simulink model "parameter_sweep_Mechanical"  (R2020a)
settings: Solver=FixedStepAuto  StartTime=0.0  StopTime=0.05  FixedStep=0.00001  RelTol=1e-3
values from neighbouring files (symbols this model uses):
  A_w = 1    [parameter_sweep_LRM_plotter.m]    (also in parameter_sweep_Mechanical_plotter.m)
  D_V = 0.00001    (= 1e-05)    [parameter_sweep_Mechanical_plotter.m]
  F_BW = 0.00001    (= 1e-05)    [parameter_sweep_Mechanical_plotter.m]
  F_C = 0.00001    (= 1e-05)    [parameter_sweep_Mechanical_plotter.m]
  G = -(Mass * 9.81)    (= -0.3924)    [parameter_sweep_Mechanical_plotter.m]
  K = 0.25    [parameter_sweep_Mechanical_plotter.m]
  K_Z = 0    [parameter_sweep_Mechanical_plotter.m]
  l_w = 1    [parameter_sweep_LRM_plotter.m]    (also in parameter_sweep_Mechanical_plotter.m)
  Ltch_End = 15    [parameter_sweep_Mechanical_plotter.m]
  Ltch_St = 12    [parameter_sweep_Mechanical_plotter.m]
  Ltch_Str = 5    [parameter_sweep_Mechanical_plotter.m]
  Mass = 0.04    [parameter_sweep_Mechanical_plotter.m]
  Mur = 1    [parameter_sweep_Mechanical_plotter.m]
  Nw = 4    [parameter_sweep_LRM_plotter.m]    (also in parameter_sweep_Mechanical_plotter.m = 300)
  R = 4.95    [parameter_sweep_LRM_plotter.m]    (also in parameter_sweep_LR_plotter.m = 7; parameter_sweep_M_plotter.m = 7; parameter_sweep_Mechanical_plotter.m = 5)
  R_Int = 0.55    [parameter_sweep_LRM_plotter.m]    (also in parameter_sweep_Mechanical_plotter.m = 0.33)
  Rel = Nw^2/ (0.004)    (= 4000)    [parameter_sweep_LRM_plotter.m]    (also in parameter_sweep_M_plotter.m = 0 + ((i-1) * 10); parameter_sweep_Mechanical_plotter.m = 0)
  Rel2 = (Nw^2)/ (0.08)    (= 1125000)    [parameter_sweep_Mechanical_plotter.m]
  V_T = 33.5    [parameter_sweep_LRM_plotter.m]    (also in parameter_sweep_LR_plotter.m = 4 + ((i-1) * 1); parameter_sweep_M_plotter.m = 350; parameter_sweep_Mechanical_plotter.m)
undefined symbols (not defined in the file or in its folder): R_Rate
libraries: nesl_utility x29, fl_lib x20, simulink x3, sdl_lib x1
settings Model: Creator=insat  LastModifiedBy=gwb15193

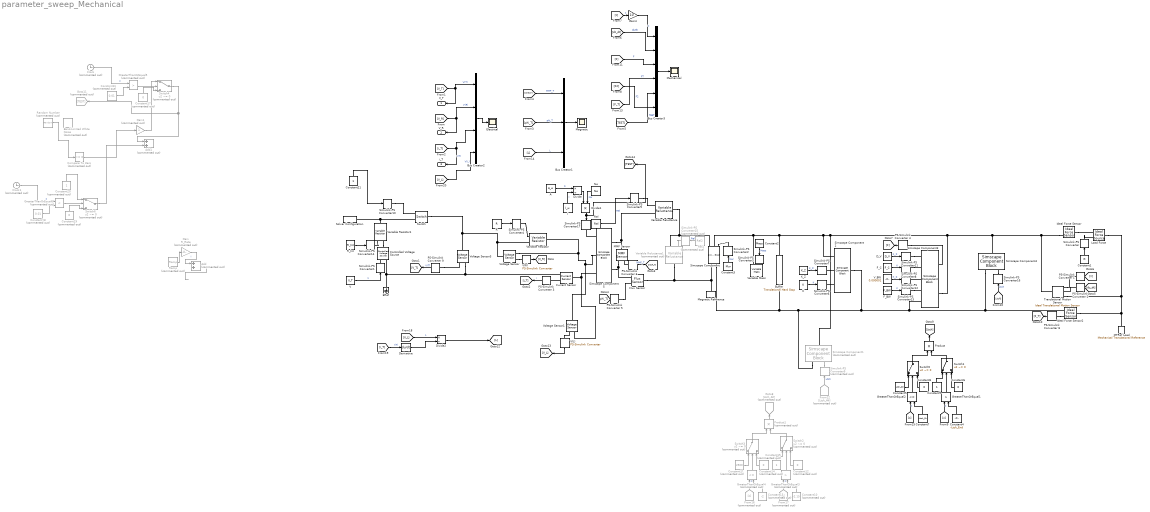
== system parameter_sweep_Mechanical ==
  A : Constant  Value=A_w
  Add : Sum  Commented=on
  Add1 : Sum  Commented=on
  Band-Limited White Noise : simulink/Sources/Band-Limited White Noise  Commented=on  Cov=[0.001]  Ts=0.00001  seed=[2334]
  Buffer : fl_lib/Mechanical/Translational Elements/Translational Hard Stop  upper_bnd=20 mm  lower_bnd=-.9 mm  stiff_up=100 N/mm  stiff_low=100 N/mm  D_up=10000000000000 s*N/mm  D_low=100 s*N/mm  model=simscape.enum.hardstop.fullundamped  transition=1 mm  v_specify=off  v_priority=None  v=0 m/s  v_nominal_specify=off  v_nominal_unit=m/s  v_nominal_value=1  f_specify=off  f_priority=None  f=0 N  f_nominal_specify=off  f_nominal_unit=N  f_nominal_value=1  x_specify=off  x_priority=High  x=0 m  x_nominal_specify=off  x_nominal_unit=m  x_nominal_value=1
  Bus Creator1 : BusCreator  Inputs=3
  Bus Creator2 : BusCreator  Inputs=4
  Bus Creator3 : BusCreator  Inputs=6
  Clock : Clock  Commented=on
  Clock1 : Clock  Commented=on
  Compare To Zero : simulink/Logic and Bit Operations/Compare To Zero  Commented=on  relop=<=  OutDataTypeStr=boolean
  Constant1 : Constant  Value=G
  Constant10 : Constant  Commented=on  Value=-2.15
  Constant11 : Constant  Commented=on  Value=2500
  Constant{12,14,17,19} (4 alike) : Constant  Commented=on  Value=0
  Constant13 : Constant  Commented=on  Value=-2
  Constant15 : Constant  Commented=on
  Constant16 : Constant  Commented=on  Value=0.01
  Constant18 : Constant  Commented=on  Value=0.01
  Constant2 : Constant  Value=Mass
  Constant20 : Constant  Commented=on
  Constant21 : Constant
  Constant3 : Constant  Value=Mur
  Constant4 : Constant  Value=-Ltch_End
  Constant5 : Constant  Value=Ltch_Str
  Constant6 : Constant  Value=0
  Constant7 : Constant  Value=-Ltch_St
  Constant8 : Constant  Value=0
  Constant9 : Constant
  Controlled Voltage Source : fl_lib/Electrical/Electrical Sources/Controlled Voltage Source
  Current Sensor : fl_lib/Electrical/Electrical Sensors/Current Sensor
  D_V : Constant  Value=D_V
  Derivative : Derivative
  Divide : Product  Inputs=*/
  Divide1 : Product  Inputs=**
  Divide2 : Product  Inputs=*/
  ERef : fl_lib/Electrical/Electrical Elements/Electrical Reference
  Electrical : Scope
  F_BW : Constant  Value=F_BW
  F_C : Constant  Value=F_C
  Flux Sensor : fl_lib/Magnetic/Magnetic Sensors/Flux Sensor
      settings: SourceProductBaseCode=SS  InternalSimscapePortConfiguration="{\"Bottom\":[],\"Left\":[{\"id\":\"N\",\"label\":\"N\",\"type\":\"foundation.magnetic.magnetic\"}],\"Right\":[{\"id\":\"PHI\",\"label\":\"\",\"type\":\"output\"},{\"id\":\"S\",\"label\":\"S\",\"type\":\"foundation.magnetic.magnetic\"}],\"Top\":[]}"
  From12 : From  Commented=on  GotoTag=Ltch_Alt
  From16 : From  Commented=on  GotoTag=z
  From17 : From  Commented=on  GotoTag=z
  Gain : Gain  Commented=on  Gain=R_Rate
  Gain1 : Gain  Commented=on
  Gain4 : Gain  Gain=10
  Goto11 : Goto  Commented=on  GotoTag=TEST
  Goto8 : Goto  Commented=on  GotoTag=Ltch_Alt
  GreaterThanOrEqual1 : RelationalOperator  Operator=>  OutDataTypeStr=boolean  ZeroCross=off  RndMeth=Simplest
  GreaterThanOrEqual2 : RelationalOperator  Operator=<=  OutDataTypeStr=boolean  ZeroCross=off  RndMeth=Simplest
  GreaterThanOrEqual3 : RelationalOperator  Commented=on  Operator=>  OutDataTypeStr=boolean  ZeroCross=off  RndMeth=Simplest
  GreaterThanOrEqual4 : RelationalOperator  Commented=on  Operator=<=  OutDataTypeStr=boolean  ZeroCross=off  RndMeth=Simplest
  GreaterThanOrEqual5 : RelationalOperator  Commented=on  Operator=>  OutDataTypeStr=boolean  ZeroCross=off  RndMeth=Simplest
  GreaterThanOrEqual6 : RelationalOperator  Commented=on  Operator=<  OutDataTypeStr=boolean  ZeroCross=off  RndMeth=Simplest
  Ideal Force Sensor : fl_lib/Mechanical/Mechanical Sensors/Ideal Force Sensor
  Ideal Force Sensor2 : fl_lib/Mechanical/Mechanical Sensors/Ideal Force Sensor
  K : Constant  Value=K
  K_Z : Constant  Value=K_Z
  Load Force : fl_lib/Mechanical/Mechanical Sources/Ideal Force Source
  MMF Sensor : fl_lib/Magnetic/Magnetic Sensors/MMF Sensor
      settings: SourceProductBaseCode=SS  InternalSimscapePortConfiguration="{\"Bottom\":[],\"Left\":[{\"id\":\"N\",\"label\":\"N\",\"type\":\"foundation.magnetic.magnetic\"}],\"Right\":[{\"id\":\"MMF\",\"label\":\"\",\"type\":\"output\"},{\"id\":\"S\",\"label\":\"S\",\"type\":\"foundation.magnetic.magnetic\"}],\"Top\":[]}"
  MTRef Load : fl_lib/Mechanical/Translational Elements/Mechanical Translational Reference
  Magnetic : Scope
  Magnetic Reference : fl_lib/Magnetic/Magnetic Elements/Magnetic Reference
      settings: SourceProductBaseCode=SS  InternalSimscapePortConfiguration="{\"Bottom\":[],\"Left\":[{\"id\":\"M\",\"label\":\"\",\"type\":\"foundation.magnetic.magnetic\"}],\"Right\":[],\"Top\":[]}"
  Mechanical : Scope
  Nw : Constant  Value=Nw
  PS-Simulink Converter 1 : nesl_utility/PS-Simulink Converter  PhysicalDomain=network_engine_domain  SubClassName=ps_output  LeftPortType=input  RightPortType=output  PseudoPeriodic=off  Frequencies=[]  Unit=mm  AffineConversion=off
  PS-Simulink Converter 2 : nesl_utility/PS-Simulink Converter  PhysicalDomain=network_engine_domain  SubClassName=ps_output  LeftPortType=input  RightPortType=output  PseudoPeriodic=off  Frequencies=[]  Unit=mm/s  AffineConversion=off
  PS-Simulink Converter 3 : nesl_utility/PS-Simulink Converter  PhysicalDomain=network_engine_domain  SubClassName=ps_output  LeftPortType=input  RightPortType=output  PseudoPeriodic=off  Frequencies=[]  Unit=A  AffineConversion=off
  PS-Simulink Converter 4 : nesl_utility/PS-Simulink Converter  PhysicalDomain=network_engine_domain  SubClassName=ps_output  LeftPortType=input  RightPortType=output  PseudoPeriodic=off  Frequencies=[]  Unit=N  AffineConversion=off
  PS-Simulink Converter 5 : nesl_utility/PS-Simulink Converter  PhysicalDomain=network_engine_domain  SubClassName=ps_output  LeftPortType=input  RightPortType=output  PseudoPeriodic=off  Frequencies=[]  Unit=Wb  AffineConversion=off
  PS-Simulink Converter 6 : nesl_utility/PS-Simulink Converter  PhysicalDomain=network_engine_domain  SubClassName=ps_output  LeftPortType=input  RightPortType=output  PseudoPeriodic=off  Frequencies=[]  Unit=A  AffineConversion=off
  PS-Simulink Converter 8 : nesl_utility/PS-Simulink Converter  PhysicalDomain=network_engine_domain  SubClassName=ps_output  LeftPortType=input  RightPortType=output  PseudoPeriodic=off  Frequencies=[]  Unit=N  AffineConversion=off
  PS-Simulink Converter 9 : nesl_utility/PS-Simulink Converter  PhysicalDomain=network_engine_domain  SubClassName=ps_output  LeftPortType=input  RightPortType=output  PseudoPeriodic=off  Frequencies=[]  Unit=V  AffineConversion=off
  Product : Product
  Product1 : Product  Commented=on
  R : Constant  Value=R
  R_Int : Constant  Value=R_Int
  Ramp : simulink/Sources/Ramp  Commented=on  slope=1  start=0.01  InitialOutput=0
  Random Number : RandomNumber  Commented=on  Mean=-30  Variance=1000  SampleTime=0.0001
  Rel : Constant  Value=Rel
  Rel1 : Constant  Commented=on  Value=Rel2
  Simscape Component : SimscapeComponentBlock  SourceFile=reluctance_force_actuator_modified  ComponentPath=reluctance_force_actuator_modified  ComponentVariants="[\"reluctance_force_actuator_modified\"]"  ComponentVariantNames="[\"reluctance_force_actuator_modified\"]"  ClassName=reluctance_force_actuator_modified  SchemaVersion=1  x0=22 mm  xbffr=1e-4 mm  CSA=1.7671 cm^2  K_contact=0.001 N/mm  D_contact=0.001 s*N/mm  mmf_specify=off  mmf_priority=None  mmf=0 A  mmf_nominal_specify=off  mmf_nominal_unit=A  mmf_nominal_value=1  phi_specify=off  phi_priority=None  phi=0 Wb  phi_nominal_specify=off  phi_nominal_unit=Wb  phi_nominal_value=1  f_specify=off  f_priority=None  f=0 N  f_nominal_specify=off  f_nominal_unit=N  f_nominal_value=1  u_specify=off  u_priority=None  u=0 m/s  u_nominal_specify=off  u_nominal_unit=m/s  u_nominal_value=1
      settings: CopyFcn=simscape.engine.sli.internal.componentblockcallback(gcbh,'COPY')  PreCopyFcn=simscape.engine.sli.internal.componentblockcallback(gcbh,'PRECOPY')  PreDeleteFcn=simscape.engine.sli.internal.componentblockcallback(gcbh,'PREDELETE')  InternalSimscapePortConfiguration="{\"Bottom\":[],\"Left\":[{\"id\":\"N\",\"label\":\"N\",\"type\":\"foundation.magnetic.magnetic\"},{\"id\":\"R\",\"label\":\"R\",\"type\":\"foundation.mechanical.translational.translational\"},{\"id\":\"mur\",\"label\":\"Mur\",\"type\":\"input\"}],\"Right\":[{\"id\":\"S\",\"label\":\"S\",\"type\":\"foundation.magnetic.magnetic\"},{\"id\":\"C\",\"label\":\"C\",\"type\":\"foundation.mechanical.translational.translational\"}],\"Top\":[]}"
      mask Type: Reluctance Force Actuator
  Simscape Component1 : SimscapeComponentBlock  Commented=on  SourceFile=damper_mod  ComponentPath=damper_mod  ComponentVariants="[\"damper_mod\"]"  ComponentVariantNames="[\"damper_mod\"]"  ClassName=damper_mod  SchemaVersion=1  v_specify=off  v_priority=None  v=0 m/s  v_nominal_specify=off  v_nominal_unit=m/s  v_nominal_value=1  f_specify=off  f_priority=None  f=0 N  f_nominal_specify=off  f_nominal_unit=N  f_nominal_value=1
      settings: CopyFcn=simscape.engine.sli.internal.componentblockcallback(gcbh,'COPY')  PreCopyFcn=simscape.engine.sli.internal.componentblockcallback(gcbh,'PRECOPY')  PreDeleteFcn=simscape.engine.sli.internal.componentblockcallback(gcbh,'PREDELETE')  InternalSimscapePortConfiguration="{\"Bottom\":[],\"Left\":[{\"id\":\"R\",\"label\":\"R\",\"type\":\"foundation.mechanical.translational.translational\"},{\"id\":\"D\",\"label\":\"Damping coefficient\",\"type\":\"input\"}],\"Right\":[{\"id\":\"C\",\"label\":\"C\",\"type\":\"foundation.mechanical.translational.translational\"}],\"Top\":[]}"
      mask Type: Translational Damper
  Simscape Component2 : SimscapeComponentBlock  SourceFile=var_trans_spring_mod  ComponentPath=var_trans_spring_mod  ComponentVariants="[\"var_trans_spring_mod\"]"  ComponentVariantNames="[\"var_trans_spring_mod\"]"  ClassName=var_trans_spring_mod  SchemaVersion=1  Kmin=1 N/m
      settings: CopyFcn=simscape.engine.sli.internal.componentblockcallback(gcbh,'COPY')  PreCopyFcn=simscape.engine.sli.internal.componentblockcallback(gcbh,'PRECOPY')  PreDeleteFcn=simscape.engine.sli.internal.componentblockcallback(gcbh,'PREDELETE')  InternalSimscapePortConfiguration="{\"Bottom\":[],\"Left\":[{\"id\":\"R\",\"label\":\"R\",\"type\":\"foundation.mechanical.translational.translational\"}],\"Right\":[{\"id\":\"K\",\"label\":\"K\",\"type\":\"input\"},{\"id\":\"Z\",\"label\":\"Z\",\"type\":\"input\"},{\"id\":\"C\",\"label\":\"C\",\"type\":\"foundation.mechanical.translational.translational\"}],\"Top\":[]}"
      mask Type: Variable Translational Spring
  Simscape Component3 : SimscapeComponentBlock  SourceFile=friction_var  ComponentPath=friction_var  ComponentVariants="[\"friction_var\"]"  ComponentVariantNames="[\"friction_var\"]"  ClassName=friction_var  SchemaVersion=1  v_specify=off  v_priority=None  v=0 m/s  v_nominal_specify=off  v_nominal_unit=m/s  v_nominal_value=1  f_specify=off  f_priority=None  f=0 N  f_nominal_specify=off  f_nominal_unit=N  f_nominal_value=1
      settings: CopyFcn=simscape.engine.sli.internal.componentblockcallback(gcbh,'COPY')  PreCopyFcn=simscape.engine.sli.internal.componentblockcallback(gcbh,'PRECOPY')  PreDeleteFcn=simscape.engine.sli.internal.componentblockcallback(gcbh,'PREDELETE')  InternalSimscapePortConfiguration="{\"Bottom\":[],\"Left\":[{\"id\":\"R\",\"label\":\"R\",\"type\":\"foundation.mechanical.translational.translational\"},{\"id\":\"brkwy_frc\",\"label\":\"F_BW\",\"type\":\"input\"},{\"id\":\"brkwy_vel\",\"label\":\"V_BW\",\"type\":\"input\"},{\"id\":\"Col_frc\",\"label\":\"F_C\",\"type\":\"input\"},{\"id\":\"visc_coef\",\"label\":\"D_V\",\"type\":\"input\"}],\"Right\":[{\"id\":\"C\",\"label\":\"C\",\"type\":\"foundation.mechanical.translational.translational\"},{\"id\":\"f_B\",\"label\":\"F\",\"type\":\"output\"}],\"Top\":[]}"
      mask Type: Translational Friction Controllable
  Simscape Component4 : SimscapeComponentBlock  SourceFile=damper_mod  ComponentPath=damper_mod  ComponentVariants="[\"damper_mod\"]"  ComponentVariantNames="[\"damper_mod\"]"  ClassName=damper_mod  SchemaVersion=1  v_specify=off  v_priority=None  v=0 m/s  v_nominal_specify=off  v_nominal_unit=m/s  v_nominal_value=1  f_specify=off  f_priority=None  f=0 N  f_nominal_specify=off  f_nominal_unit=N  f_nominal_value=1
      settings: CopyFcn=simscape.engine.sli.internal.componentblockcallback(gcbh,'COPY')  PreCopyFcn=simscape.engine.sli.internal.componentblockcallback(gcbh,'PRECOPY')  PreDeleteFcn=simscape.engine.sli.internal.componentblockcallback(gcbh,'PREDELETE')  InternalSimscapePortConfiguration="{\"Bottom\":[],\"Left\":[{\"id\":\"R\",\"label\":\"R\",\"type\":\"foundation.mechanical.translational.translational\"},{\"id\":\"D\",\"label\":\"Damping coefficient\",\"type\":\"input\"}],\"Right\":[{\"id\":\"C\",\"label\":\"C\",\"type\":\"foundation.mechanical.translational.translational\"}],\"Top\":[]}"
      mask Type: Translational Damper
  Simscape Component5 : SimscapeComponentBlock  SourceFile=electromagenetic_converter_mod  ComponentPath=electromagenetic_converter_mod  ComponentVariants="[\"electromagenetic_converter_mod\"]"  ComponentVariantNames="[\"electromagenetic_converter_mod\"]"  ClassName=electromagenetic_converter_mod  SchemaVersion=1  i_specify=off  i_priority=None  i=0 A  i_nominal_specify=off  i_nominal_unit=A  i_nominal_value=1  v_specify=off  v_priority=None  v=0 V  v_nominal_specify=off  v_nominal_unit=V  v_nominal_value=1  mmf_specify=off  mmf_priority=None  mmf=0 A  mmf_nominal_specify=off  mmf_nominal_unit=A  mmf_nominal_value=1  phi_specify=off  phi_priority=High  phi=0 Wb  phi_nominal_specify=off  phi_nominal_unit=Wb  phi_nominal_value=1
      settings: CopyFcn=simscape.engine.sli.internal.componentblockcallback(gcbh,'COPY')  PreCopyFcn=simscape.engine.sli.internal.componentblockcallback(gcbh,'PRECOPY')  PreDeleteFcn=simscape.engine.sli.internal.componentblockcallback(gcbh,'PREDELETE')  InternalSimscapePortConfiguration="{\"Bottom\":[],\"Left\":[{\"id\":\"p\",\"label\":\"+\",\"type\":\"foundation.electrical.electrical\"},{\"id\":\"n\",\"label\":\"-\",\"type\":\"foundation.electrical.electrical\"},{\"id\":\"Nw\",\"label\":\"Number of winding turns\",\"type\":\"input\"}],\"Right\":[{\"id\":\"N\",\"label\":\"N\",\"type\":\"foundation.magnetic.magnetic\"},{\"id\":\"S\",\"label\":\"S\",\"type\":\"foundation.magnetic.magnetic\"}],\"Top\":[]}"
      mask Type: Electromagnetic Converter
  Simulink-PS Converter{,1..8,10..14,16..17} (16 alike) : nesl_utility/Simulink-PS Converter  PhysicalDomain=network_engine_domain  SubClassName=ps_input  LeftPortType=input  RightPortType=output  PseudoPeriodic=off  Frequencies=[]  NoiseDistribution=none  NoiseParameters=[]  Unit=1  AffineConversion=off  FilteringAndDerivatives=zero  SimscapeFilterOrder=1  InputFilterTimeConstant=.001  UdotUserProvided=0
  Simulink-PS Converter15 : nesl_utility/Simulink-PS Converter  Commented=on  PhysicalDomain=network_engine_domain  SubClassName=ps_input  LeftPortType=input  RightPortType=output  PseudoPeriodic=off  Frequencies=[]  NoiseDistribution=none  NoiseParameters=[]  Unit=1  AffineConversion=off  FilteringAndDerivatives=zero  SimscapeFilterOrder=1  InputFilterTimeConstant=.001  UdotUserProvided=0
  Simulink-PS Converter9 : nesl_utility/Simulink-PS Converter  Commented=on  PhysicalDomain=network_engine_domain  SubClassName=ps_input  LeftPortType=input  RightPortType=output  PseudoPeriodic=off  Frequencies=[]  NoiseDistribution=none  NoiseParameters=[]  Unit=1  AffineConversion=off  FilteringAndDerivatives=zero  SimscapeFilterOrder=1  InputFilterTimeConstant=.001  UdotUserProvided=0
  Solver Configuration : nesl_utility/Solver Configuration  PhysicalDomain=network_engine_domain  SubClassName=solver  LeftPortType=input  RightPortType=generic  Tones=[]  Harmonics=[]  SimulateNoise=off  Profile=off  UseLocalSampling=off  EnableSwitchedLinearOptims=on  FrequencyDomain=off  UseCCode=off  RelTol=0.001  AbsTol=1e-06  MinStep=1e-09  ToWorkspace=off  RevertToSquareIcSolve=off  NumHomotopyIterations=100  PhasorMode=off  PhasorModeNumHarmonics=1  DoDC=off  ResidualTolerance=1e-9  UseLocalSolver=off  LocalSolverChoice=NE_BACKWARD_EULER_ADVANCER  LocalSolverSampleTime=.001  DoFixedCost=off  MaxNonlinIter=3  MaxModeIter=2  LinearAlgebra=auto  EquationFormulation=NE_TIME_EF  DelaysMemoryBudget=1024  AutomaticFiltering=on  FilteringTimeConstant=0.0001  PartitionStorageMethod=AS_NEEDED  PartitionMemoryBudget=1024  PartitionMethod=FAST
  Switch : fl_lib/Electrical/Electrical Elements/Switch  R_closed=0.01 Ohm  G_open=1e-8 1/Ohm  Threshold=0  i_specify=off  i_priority=None  i=0 A  i_nominal_specify=off  i_nominal_unit=A  i_nominal_value=1  v_specify=off  v_priority=None  v=0 V  v_nominal_specify=off  v_nominal_unit=V  v_nominal_value=1
  Switch1 : Switch  Criteria=u2 ~= 0  ZeroCross=off
  Switch{2..4,6} (4 alike) : Switch  Commented=on  Criteria=u2 ~= 0  ZeroCross=off
  Switch5 : Switch  Criteria=u2 ~= 0  ZeroCross=off
  Translational Motion Sensor : fl_lib/Mechanical/Mechanical Sensors/Ideal Translational Motion Sensor  offset=0 mm
  V : Constant  Value=V_T
  V(L) : nesl_utility/PS-Simulink Converter  PhysicalDomain=network_engine_domain  SubClassName=ps_output  LeftPortType=input  RightPortType=output  PseudoPeriodic=off  Frequencies=[]  Unit=V  AffineConversion=off
  V(R) : nesl_utility/PS-Simulink Converter  PhysicalDomain=network_engine_domain  SubClassName=ps_output  LeftPortType=input  RightPortType=output  PseudoPeriodic=off  Frequencies=[]  Unit=V  AffineConversion=off
  V_BW : Constant  Value=0.000001
  Variable Mass : sdl_lib/Inertias & Loads/Variable Mass  minimum_mass=0.0001 kg  p_specify=off  p_priority=High  p=0 m*kg/s  p_nominal_specify=off  p_nominal_unit=m*kg/s  p_nominal_value=1
      settings: SourceProductBaseCode=LD  InternalSimscapePortConfiguration="{\"Bottom\":[],\"Left\":[{\"id\":\"M\",\"label\":\"\",\"type\":\"input\"},{\"id\":\"A\",\"label\":\"\",\"type\":\"foundation.mechanical.translational.translational\"}],\"Right\":[],\"Top\":[]}"
  Variable Reluctance : fl_lib/Magnetic/Magnetic Elements/Variable Reluctance  Xmin=0.000000001 m  CSA=1 m^2  mur=1  phi_specify=off  phi_priority=None  phi=0 Wb  phi_nominal_specify=off  phi_nominal_unit=Wb  phi_nominal_value=1  mmf_specify=off  mmf_priority=None  mmf=0 A  mmf_nominal_specify=off  mmf_nominal_unit=A  mmf_nominal_value=1
      settings: SourceProductBaseCode=SS  InternalSimscapePortConfiguration="{\"Bottom\":[],\"Left\":[{\"id\":\"N\",\"label\":\"N\",\"type\":\"foundation.magnetic.magnetic\"},{\"id\":\"X\",\"label\":\"\",\"type\":\"input\"}],\"Right\":[{\"id\":\"S\",\"label\":\"S\",\"type\":\"foundation.magnetic.magnetic\"}],\"Top\":[]}"
  Variable Reluctance1 : fl_lib/Magnetic/Magnetic Elements/Variable Reluctance  Commented=on  Xmin=0.000000001 m  CSA=1 m^2  mur=1  phi_specify=off  phi_priority=None  phi=0 Wb  phi_nominal_specify=off  phi_nominal_unit=Wb  phi_nominal_value=1  mmf_specify=off  mmf_priority=None  mmf=0 A  mmf_nominal_specify=off  mmf_nominal_unit=A  mmf_nominal_value=1
      settings: SourceProductBaseCode=SS  InternalSimscapePortConfiguration="{\"Bottom\":[],\"Left\":[{\"id\":\"N\",\"label\":\"N\",\"type\":\"foundation.magnetic.magnetic\"},{\"id\":\"X\",\"label\":\"\",\"type\":\"input\"}],\"Right\":[{\"id\":\"S\",\"label\":\"S\",\"type\":\"foundation.magnetic.magnetic\"}],\"Top\":[]}"
  Variable Resistor : fl_lib/Electrical/Electrical Elements/Variable Resistor  Rmin=0 Ohm  i_specify=off  i_priority=None  i=0 A  i_nominal_specify=off  i_nominal_unit=A  i_nominal_value=1  v_specify=off  v_priority=None  v=0 V  v_nominal_specify=off  v_nominal_unit=V  v_nominal_value=1
  Variable Resistor1 : fl_lib/Electrical/Electrical Elements/Variable Resistor  Rmin=0 Ohm  i_specify=off  i_priority=None  i=0 A  i_nominal_specify=off  i_nominal_unit=A  i_nominal_value=1  v_specify=off  v_priority=None  v=0 V  v_nominal_specify=off  v_nominal_unit=V  v_nominal_value=1
  Voltage Sensor : fl_lib/Electrical/Electrical Sensors/Voltage Sensor
  Voltage Sensor1 : fl_lib/Electrical/Electrical Sensors/Voltage Sensor
  Voltage Sensor3 : fl_lib/Electrical/Electrical Sensors/Voltage Sensor
  l : Constant  Value=l_w
  V_T : Outport  SignalName=V_T
  V_R : Outport  Port=2  SignalName=V_R
  i_T : Outport  Port=3  SignalName=i_T
  wires:
  V/1 -> Simulink-PS Converter1/1  "V"
  V(R)/1 -> [V_R]
  PS-Simulink Converter 3/1 -> [i_T]  "i"
  PS-Simulink Converter 9/1 -> [V_T]  "V(T)"
  Bus Creator2/1 -> Electrical/1
  [i_T] -> i_T/1, Bus Creator2/3  "i(T)"
  [V_T] -> V_T/1, Bus Creator2/1  "V(T)"
  [V_R] -> V_R/1, Bus Creator2/2  "V(R)"
  PS-Simulink Converter 5/1 -> [phi_T]
  PS-Simulink Converter 6/1 -> [MMF_T]  "MMF_T"
  [MMF_T] -> Bus Creator1/1  "MMF_T"
  [phi_T] -> Bus Creator1/2  "phi_T"
  Bus Creator1/1 -> Magnetic/1
  [L] -> Bus Creator1/3  "L"
  [F] -> Bus Creator3/3  "F"
  [F_T] -> Bus Creator3/4  "FT"
  [F2] -> Bus Creator3/6  "F2"
  Gain4/1 -> Bus Creator3/1  "z"
  [z] -> Gain4/1  "z"
  [dz_dt] -> Bus Creator3/2  "dz/dt"
  Bus Creator3/1 -> Mechanical/1
  [TEST] -> Bus Creator3/5  "TEST"
  Rel/1 -> Simulink-PS Converter5/1  "Rel"
  PS-Simulink Converter 4/1 -> [F]
  PS-Simulink Converter 8/1 -> [F_T]
  PS-Simulink Converter 2/1 -> [dz_dt]
  PS-Simulink Converter 1/1 -> [z]
  Constant2/1 -> Simulink-PS Converter3/1  "Mass"
  Constant3/1 -> Simulink-PS Converter2/1  "Mur"
  K_Z/1 -> Simulink-PS Converter7/1  "K_Z"
  K/1 -> Simulink-PS Converter6/1  "K"
  D_V/1 -> Simulink-PS Converter11/1  "K_Z"
  V_BW/1 -> Simulink-PS Converter12/1  "K_Z"
  F_C/1 -> Simulink-PS Converter8/1  "K"
  F_BW/1 -> Simulink-PS Converter13/1  "K"
  Product/1 -> [Ltch]
  [z] -> GreaterThanOrEqual1/1  "z"
  Constant4/1 -> GreaterThanOrEqual1/2
  Constant8/1 -> Switch5/3
  Switch1/1 -> Product/2
  Switch5/1 -> Product/1
  Constant7/1 -> GreaterThanOrEqual2/2
  Constant9/1 -> Switch1/1
  GreaterThanOrEqual2/1 -> Switch5/2
  GreaterThanOrEqual1/1 -> Switch1/2
  Constant6/1 -> Switch1/3
  [z] -> GreaterThanOrEqual2/1  "z"
  Constant5/1 -> Switch5/1
  [Ltch] -> Simulink-PS Converter16/1  "Ltch"
  From12/1 -> Simulink-PS Converter9/1  "Ltch"
  Constant15/1 -> Switch2/1
  Constant13/1 -> GreaterThanOrEqual4/2
  Switch3/1 -> Product1/1
  Constant14/1 -> Switch3/3
  Constant10/1 -> GreaterThanOrEqual3/2
  From17/1 -> GreaterThanOrEqual3/1  "z"
  Product1/1 -> Goto8/1
  Constant11/1 -> Switch3/1
  Constant12/1 -> Switch2/3
  GreaterThanOrEqual4/1 -> Switch3/2
  Switch2/1 -> Product1/2
  GreaterThanOrEqual3/1 -> Switch2/2
  From16/1 -> GreaterThanOrEqual4/1  "z"
  Constant1/1 -> Simulink-PS Converter/1
  Add/1 -> ?
  Ramp/1 -> Gain/1
  Gain/1 -> Add/1  "i"
  ? -> Add/2  "R"
  R/1 -> Simulink-PS Converter4/1
  Constant16/1 -> GreaterThanOrEqual5/2
  Clock/1 -> GreaterThanOrEqual5/1  "z"
  Compare To Zero/1 -> Gain1/1
  Gain1/1 -> Switch4/1
  Random Number/1 -> Compare To Zero/1
  GreaterThanOrEqual5/1 -> Switch4/2
  Switch6/1 -> Add1/2
  Constant17/1 -> Switch4/3
  Switch4/1 -> Add1/1, Goto11/1
  Constant19/1 -> Switch6/3
  Clock1/1 -> GreaterThanOrEqual6/1  "z"
  Constant18/1 -> GreaterThanOrEqual6/2
  GreaterThanOrEqual6/1 -> Switch6/2
  Constant20/1 -> Switch6/1
  Constant21/1 -> Simulink-PS Converter10/1
  R_Int/1 -> Simulink-PS Converter14/1
  Rel1/1 -> Simulink-PS Converter15/1  "Rel"
  Divide2/1 -> [L]
  V(L)/1 -> [V_L]
  [V_L] -> Divide2/1  "L"
  Derivative/1 -> Divide2/2
  [i_T] -> Derivative/1  "i(T)"
  [V_L] -> Bus Creator2/4  "V(L)"
  l/1 -> Divide/2  "l"
  Nw/1 -> Divide1/2  "Nw"
  Divide1/1 -> [TEST], Simulink-PS Converter17/1
  Divide/1 -> Divide1/1
  A/1 -> Divide/1  "A"
  connections:
  ERef/LConn1 -- Current Sensor/RConn2 -- Voltage Sensor3/RConn2 -- Controlled Voltage Source/RConn2
  Voltage Sensor/LConn1 -- Variable Resistor/LConn2 -- Switch/LConn1 -- Voltage Sensor3/LConn1
  Voltage Sensor/RConn2 -- Variable Resistor/RConn1 -- Simscape Component5/LConn2 -- Voltage Sensor1/LConn1
  Current Sensor/RConn1 -- PS-Simulink Converter 3/LConn1
  Voltage Sensor/RConn1 -- V(R)/LConn1
  Simulink-PS Converter1/RConn1 -- Controlled Voltage Source/RConn1
  PS-Simulink Converter 9/LConn1 -- Voltage Sensor3/RConn1
  Simulink-PS Converter4/RConn1 -- Variable Resistor/LConn1
  MMF Sensor/RConn2 -- Flux Sensor/RConn2 -- Simscape Component5/RConn1
  PS-Simulink Converter 5/LConn1 -- Flux Sensor/RConn1
  Simulink-PS Converter5/RConn1 -- Variable Reluctance/LConn2
  PS-Simulink Converter 6/LConn1 -- MMF Sensor/RConn1
  Current Sensor/LConn1 -- Simscape Component5/LConn1 -- Voltage Sensor1/RConn2
  Magnetic Reference/LConn1 -- Flux Sensor/LConn1 -- Variable Reluctance1/RConn1 -- Simscape Component/RConn1
  Ideal Force Sensor2/RConn1 -- Simscape Component3/LConn1 -- Simscape Component2/LConn1 -- Simscape Component1/LConn1 -- Simscape Component/RConn2 -- Buffer/LConn1 -- Simscape Component4/LConn1
  Translational Motion Sensor/RConn1 -- Load Force/LConn1 -- MTRef Load/LConn1 -- Ideal Force Sensor2/LConn1
  Ideal Force Sensor/RConn1 -- Simscape Component1/RConn1 -- Simscape Component2/RConn3 -- Buffer/RConn1 -- Simscape Component/LConn2 -- Variable Mass/LConn2 -- Simscape Component3/RConn1 -- Simscape Component4/RConn1 -- Translational Motion Sensor/LConn1
  Translational Motion Sensor/RConn3 -- PS-Simulink Converter 1/LConn1
  Ideal Force Sensor/LConn1 -- Load Force/RConn2
  PS-Simulink Converter 8/LConn1 -- Ideal Force Sensor2/RConn2
  Simulink-PS Converter/RConn1 -- Load Force/RConn1
  PS-Simulink Converter 2/LConn1 -- Translational Motion Sensor/RConn2
  Simulink-PS Converter3/RConn1 -- Variable Mass/LConn1
  Simulink-PS Converter2/RConn1 -- Simscape Component/LConn3
  Simscape Component2/RConn1 -- Simulink-PS Converter6/RConn1
  Simscape Component2/RConn2 -- Simulink-PS Converter7/RConn1
  Simulink-PS Converter11/RConn1 -- Simscape Component3/LConn5
  Simulink-PS Converter13/RConn1 -- Simscape Component3/LConn2
  Simulink-PS Converter8/RConn1 -- Simscape Component3/LConn4
  Simscape Component3/LConn3 -- Simulink-PS Converter12/RConn1
  PS-Simulink Converter 4/LConn1 -- Simscape Component3/RConn2
  Simscape Component4/LConn2 -- Simulink-PS Converter16/RConn1
  Simscape Component1/LConn2 -- Simulink-PS Converter9/RConn1
  Variable Resistor1/LConn2 -- Controlled Voltage Source/LConn1
  Simulink-PS Converter10/RConn1 -- Switch/RConn1
  Switch/RConn2 -- Variable Resistor1/RConn1 -- Solver Configuration/RConn1
  Simulink-PS Converter14/RConn1 -- Variable Resistor1/LConn1
  Simulink-PS Converter15/RConn1 -- Variable Reluctance1/LConn2
  MMF Sensor/LConn1 -- Simscape Component5/RConn2 -- Variable Reluctance/LConn1
  Voltage Sensor1/RConn1 -- V(L)/LConn1
  Simscape Component/LConn1 -- Variable Reluctance1/LConn1 -- Variable Reluctance/RConn1
  Simscape Component5/LConn3 -- Simulink-PS Converter17/RConn1
